simulink model "FlatEarth_ports_MATLAB5"  (Simulink 2.20)
settings: Solver=ode45  StartTime=0.0  StopTime=10.0  RelTol=1e-3
undefined symbols (not defined in the file or in its folder): constant, xIC
settings Model: ConsistencyChecking=off  RTWPlaceOutputsASAP=off

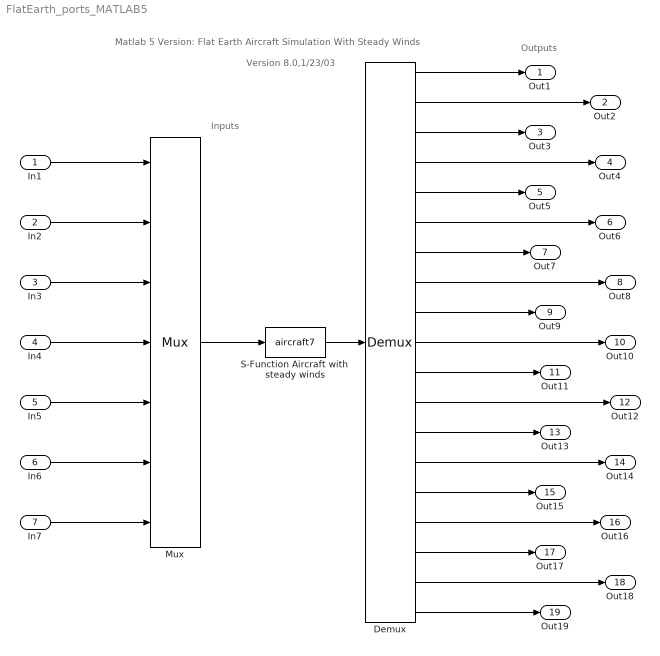
== system FlatEarth_ports_MATLAB5 ==
  note: Matlab 5 Version: Flat Earth Aircraft Simulation With Steady Winds
  note: Version 8.0,1/23/03
  note: Inputs
  note: Outputs
  In1 : Inport  Port=1  PortWidth=-1  SampleTime=-1
  In2 : Inport  Port=2  PortWidth=-1  SampleTime=-1
  In3 : Inport  Port=3  PortWidth=-1  SampleTime=-1
  In4 : Inport  Port=4  PortWidth=-1  SampleTime=-1
  In5 : Inport  Port=5  PortWidth=-1  SampleTime=-1
  In6 : Inport  Port=6  PortWidth=-1  SampleTime=-1
  In7 : Inport  Port=7  PortWidth=-1  SampleTime=-1
  Demux : Demux  Outputs=19
  Mux : Mux  Inputs=7
  S-Function Aircraft with  steady winds : S-Function  FunctionName=aircraft7  Parameters=constant,xIC  PortCounts=[]  SFunctionModules=''
  Out1 : Outport  Port=1
  Out2 : Outport  Port=2
  Out3 : Outport  Port=3
  Out4 : Outport  Port=4
  Out5 : Outport  Port=5
  Out6 : Outport  Port=6
  Out7 : Outport  Port=7
  Out8 : Outport  Port=8
  Out9 : Outport  Port=9
  Out10 : Outport  Port=10
  Out11 : Outport  Port=11
  Out12 : Outport  Port=12
  Out13 : Outport  Port=13
  Out14 : Outport  Port=14
  Out15 : Outport  Port=15
  Out16 : Outport  Port=16
  Out17 : Outport  Port=17
  Out18 : Outport  Port=18
  Out19 : Outport  Port=19
  wires:
  In1/1 -> Mux/1
  In2/1 -> Mux/2
  In3/1 -> Mux/3
  In4/1 -> Mux/4
  In5/1 -> Mux/5
  In6/1 -> Mux/6
  In7/1 -> Mux/7
  Mux/1 -> S-Function Aircraft with  steady winds/1
  S-Function Aircraft with  steady winds/1 -> Demux/1
  Demux/1 -> Out1/1
  Demux/2 -> Out2/1
  Demux/3 -> Out3/1
  Demux/4 -> Out4/1
  Demux/5 -> Out5/1
  Demux/6 -> Out6/1
  Demux/7 -> Out7/1
  Demux/8 -> Out8/1
  Demux/9 -> Out9/1
  Demux/10 -> Out10/1
  Demux/11 -> Out11/1
  Demux/12 -> Out12/1
  Demux/13 -> Out13/1
  Demux/14 -> Out14/1
  Demux/15 -> Out15/1
  Demux/16 -> Out16/1
  Demux/18 -> Out18/1
  Demux/17 -> Out17/1
  Demux/19 -> Out19/1
